simulink model "Tugas_Akhir"  (R2024a)
settings: Solver=VariableStepAuto  StartTime=0.0  StopTime=10.0  RelTol=1e-3
settings Model: Creator=Lenovo  LastModifiedBy=Lenovo

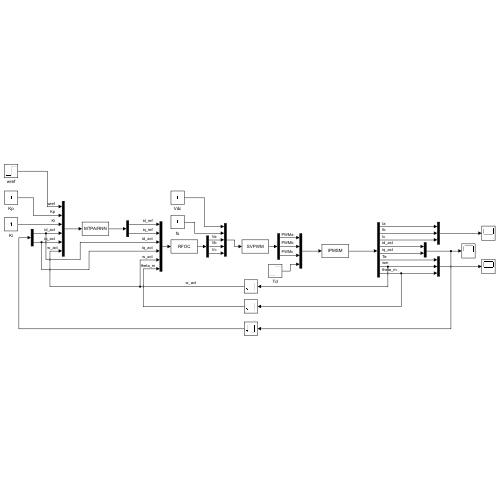
[thumbnail: Simulink's stored preview of the top-level diagram]
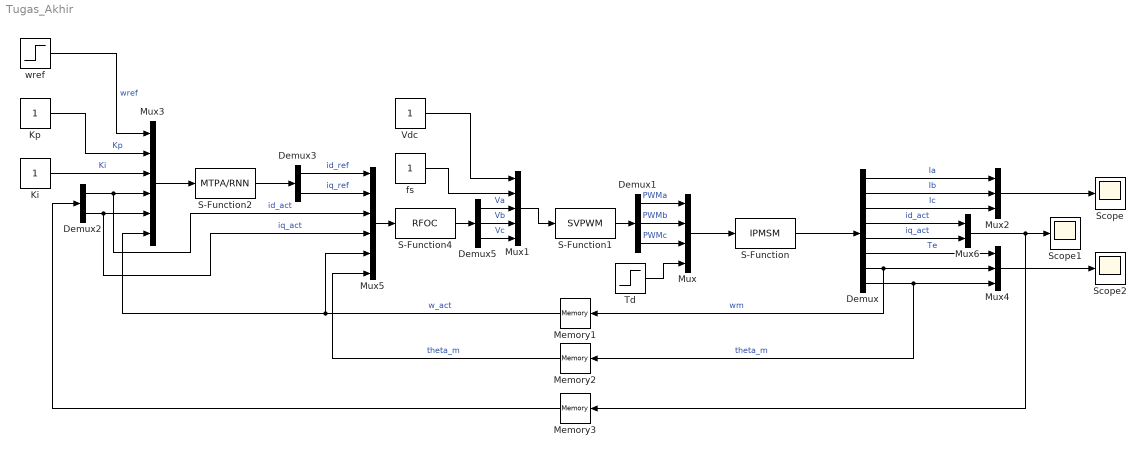
== system Tugas_Akhir ==
  Demux : Demux  Outputs=8
  Demux1 : Demux  Outputs=3
  Demux2 : Demux  Outputs=2
  Demux3 : Demux  Outputs=2
  Demux5 : Demux  Outputs=3
  Ki : Constant
  Kp : Constant
  Memory1 : Memory
  Memory2 : Memory
  Memory3 : Memory
  Mux : Mux
  Mux1 : Mux  Inputs=5
  Mux2 : Mux  Inputs=3
  Mux3 : Mux  Inputs=6
  Mux4 : Mux  Inputs=3
  Mux5 : Mux  Inputs=6
  Mux6 : Mux  Inputs=2
  S-Function : S-Function  FunctionName=IPMSM  SFunctionDeploymentMode=off  EnableBusSupport=off
  S-Function1 : S-Function  FunctionName=SVPWM  SFunctionDeploymentMode=off  EnableBusSupport=off
  S-Function2 : S-Function  FunctionName=MTPA/RNN  SFunctionDeploymentMode=off  EnableBusSupport=off
  S-Function4 : S-Function  FunctionName=RFOC  SFunctionDeploymentMode=off  EnableBusSupport=off
  Scope : Scope
  Scope1 : Scope
  Scope2 : Scope
  Td : Step  SampleTime=0
  Vdc : Constant
  fs : Constant
  wref : Step  SampleTime=0
  wires:
  S-Function/1 -> Demux/1
  Mux/1 -> S-Function/1
  Demux1/1 -> Mux/1  "PWMa"
  Demux1/2 -> Mux/2  "PWMb"
  Demux1/3 -> Mux/3  "PWMc"
  Td/1 -> Mux/4
  Mux1/1 -> S-Function1/1
  Demux/1 -> Mux2/1  "Ia"
  Demux/2 -> Mux2/2  "Ib"
  Demux/3 -> Mux2/3  "Ic"
  Mux2/1 -> Scope/1
  S-Function2/1 -> Demux3/1
  Mux3/1 -> S-Function2/1
  wref/1 -> Mux3/1  "wref"
  Kp/1 -> Mux3/2  "Kp"
  Ki/1 -> Mux3/3  "Ki"
  Demux/5 -> Mux6/2  "iq_act"
  Demux3/1 -> Mux5/1  "id_ref"
  Demux3/2 -> Mux5/2  "iq_ref"
  Mux5/1 -> S-Function4/1
  S-Function4/1 -> Demux5/1
  Demux5/2 -> Mux1/4  "Vb"
  Demux5/1 -> Mux1/3  "Va"
  Demux5/3 -> Mux1/5  "Vc"
  S-Function1/1 -> Demux1/1
  Memory1/1 -> Mux5/5, Mux3/6  "w_act"
  Demux/4 -> Mux6/1  "id_act"
  Demux/6 -> Mux4/1  "Te"
  Mux6/1 -> Scope1/1, Memory3/1
  Memory2/1 -> Mux5/6  "theta_m"
  Demux/7 -> Mux4/2, Memory1/1  "wm"
  Demux/8 -> Mux4/3, Memory2/1  "theta_m"
  Demux2/1 -> Mux3/4, Mux5/3  "id_act"
  Demux2/2 -> Mux5/4, Mux3/5  "iq_act"
  Mux4/1 -> Scope2/1
  Memory3/1 -> Demux2/1
  Vdc/1 -> Mux1/1
  fs/1 -> Mux1/2
